simulink model "question8_2_simulink"  (R2025b)
settings: Solver=VariableStepAuto  StartTime=0.0  StopTime=10  RelTol=1e-3
settings Model: Creator=artes  LastModifiedBy=artes

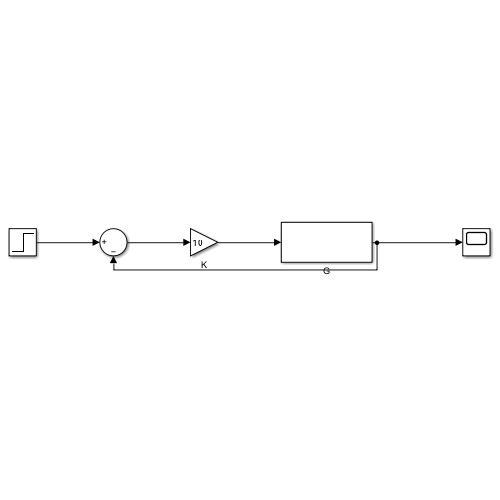
[thumbnail: Simulink's stored preview of the top-level diagram]
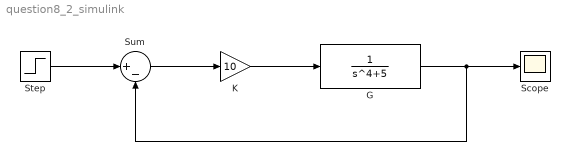
== system question8_2_simulink ==
  G : TransferFcn  Denominator=[1 0 0 0 5]
  K : Gain  Gain=10
  Scope : Scope
  Step : Step  SampleTime=0
  Sum : Sum  Inputs=|+-
  wires:
  Step/1 -> Sum/1
  Sum/1 -> K/1
  K/1 -> G/1
  G/1 -> Scope/1, Sum/2
